simulink model "sppvt_control_model"  (R2024b)
settings: Solver=FixedStepDiscrete  StartTime=0  StopTime=inf  FixedStep=0.05  RelTol=1e-3
undefined symbols (not defined in the file or in its folder): f
libraries: instrumentlib x2
settings Model: Creator=ZhaoY  LastModifiedBy=aiden
settings DataIOCC: ExternalInput=[external_input_data]  SaveFormat=StructureWithTime

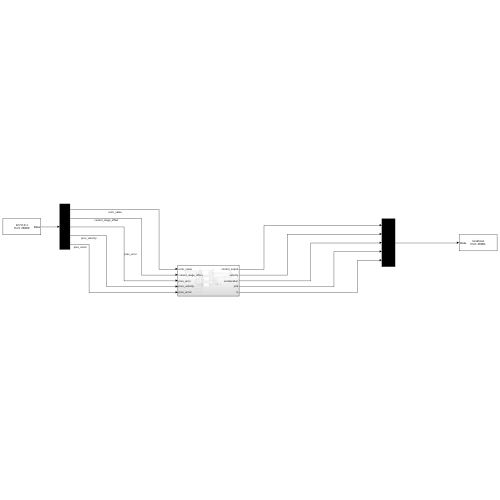
[thumbnail: Simulink's stored preview of the top-level diagram]
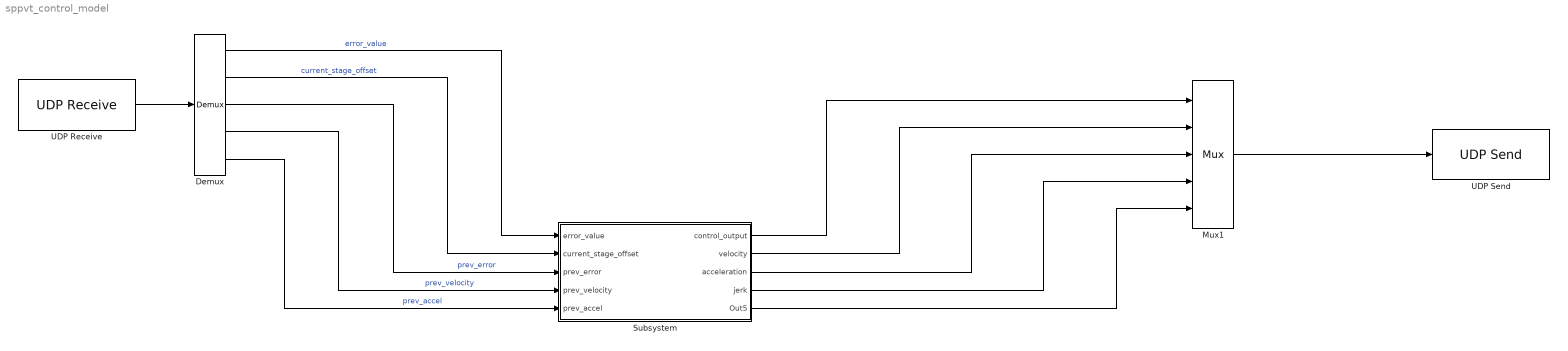
== system sppvt_control_model ==
  Demux : Demux  Outputs=5
  Mux1 : Mux  Inputs=5
  Subsystem : Subsystem
  UDP Receive : instrumentlib/UDP Receive  LocalAddress=127.0.0.1  LocalPort=26000  EnablePortSharing=off  Host=localhost  Port=9091  GetLatestData=on  DataSize=[ 5, 1 ]  DataType=double  ASCIIFormatting=%f,  Terminator=LF  CustomTerminator=10  ByteOrder=little-endian  EnableBlockingMode=on  Timeout=20  SampleTime=-1  SimulateUsing=Interpreted execution
  UDP Send : instrumentlib/UDP Send  Host=localhost  Port=26001  LocalAddress=0.0.0.0  LocalPort=26001  EnablePortSharing=on  OutputDatagramPacketSize=512  ByteOrder=little-endian  EnableBlockingMode=off  SimulateUsing=Interpreted execution
  wires:
  UDP Receive/1 -> Demux/1
  Mux1/1 -> UDP Send/1
  Demux/1 -> Subsystem/1(error_value)  "error_value"
  Demux/2 -> Subsystem/2(current_stage_offset)  "current_stage_offset"
  Demux/3 -> Subsystem/3(prev_error)  "prev_error"
  Demux/4 -> Subsystem/4(prev_velocity)  "prev_velocity"
  Demux/5 -> Subsystem/5(prev_accel)  "prev_accel"
  Subsystem/1(control_output) -> Mux1/1
  Subsystem/2(velocity) -> Mux1/2
  Subsystem/3(acceleration) -> Mux1/3
  Subsystem/4(jerk) -> Mux1/4
  Subsystem/5(Out5) -> Mux1/5

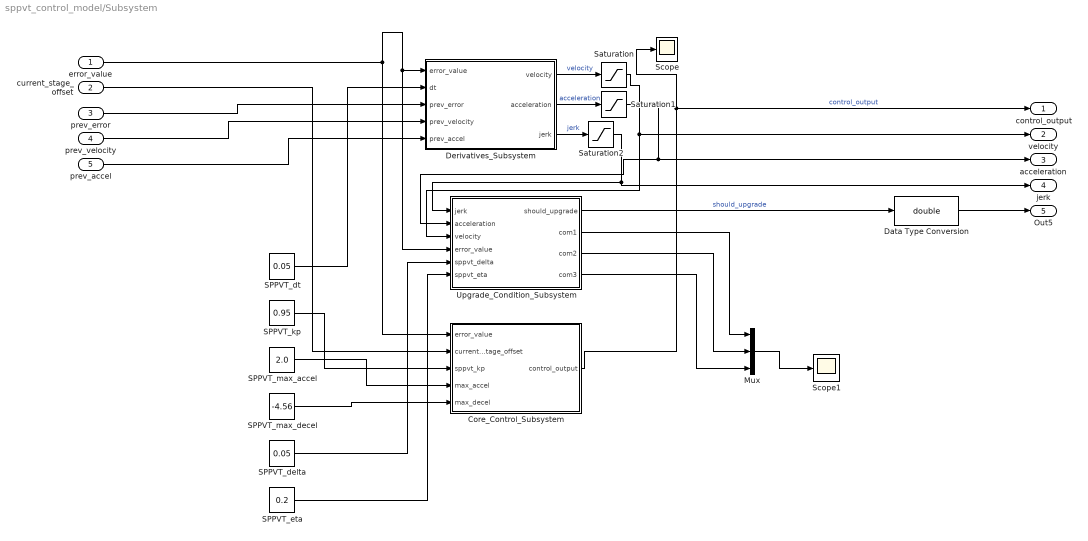
== system sppvt_control_model/Subsystem ==
  error_value : Inport
  current_stage_offset : Inport  Port=2
  prev_error : Inport  Port=3
  prev_velocity : Inport  Port=4
  prev_accel : Inport  Port=5
  Core_Control_Subsystem : Subsystem
  Data Type Conversion : DataTypeConversion  OutDataTypeStr=double  SaturateOnIntegerOverflow=off  RndMeth=Floor
  Derivatives_Subsystem : Subsystem
  Mux : Mux  Inputs=3
  SPPVT_delta : Constant  Value=0.05
  SPPVT_dt : Constant  Value=0.05
  SPPVT_eta : Constant  Value=0.2
  SPPVT_kp : Constant  Value=0.95
  SPPVT_max_accel : Constant  Value=2.0
  SPPVT_max_decel : Constant  Value=-4.56
  Saturation : Saturate  UpperLimit=5000.0  LowerLimit=-5000.0
  Saturation1 : Saturate  UpperLimit=10000.0  LowerLimit=-10000.0
  Saturation2 : Saturate  UpperLimit=20000.0  LowerLimit=-20000.0
  Scope : Scope
  Scope1 : Scope
  Upgrade_Condition_Subsystem : Subsystem
  control_output : Outport
  velocity : Outport  Port=2
  acceleration : Outport  Port=3
  jerk : Outport  Port=4
  Out5 : Outport  Port=5
  wires:
  Upgrade_Condition_Subsystem/2(com1) -> Mux/1
  Derivatives_Subsystem/3(jerk) -> Saturation2/1  "jerk"
  SPPVT_kp/1 -> Core_Control_Subsystem/3(sppvt_kp)
  Derivatives_Subsystem/2(acceleration) -> Saturation1/1  "acceleration"
  Derivatives_Subsystem/1(velocity) -> Saturation/1  "velocity"
  Core_Control_Subsystem/1(control_output) -> control_output/1, Scope/1  "control_output"
  current_stage_offset/1 -> Core_Control_Subsystem/2(current_stage_offset)
  Saturation2/1 -> jerk/1, Upgrade_Condition_Subsystem/1(jerk)
  Data Type Conversion/1 -> Out5/1
  prev_error/1 -> Derivatives_Subsystem/3(prev_error)
  Saturation/1 -> velocity/1, Upgrade_Condition_Subsystem/3(velocity)
  prev_velocity/1 -> Derivatives_Subsystem/4(prev_velocity)
  SPPVT_max_accel/1 -> Core_Control_Subsystem/4(max_accel)
  Upgrade_Condition_Subsystem/1(should_upgrade) -> Data Type Conversion/1  "should_upgrade"
  prev_accel/1 -> Derivatives_Subsystem/5(prev_accel)
  SPPVT_dt/1 -> Derivatives_Subsystem/2(dt)
  Upgrade_Condition_Subsystem/3(com2) -> Mux/2
  SPPVT_eta/1 -> Upgrade_Condition_Subsystem/6(sppvt_eta)
  SPPVT_delta/1 -> Upgrade_Condition_Subsystem/5(sppvt_delta)
  Saturation1/1 -> acceleration/1, Upgrade_Condition_Subsystem/2(acceleration)
  Upgrade_Condition_Subsystem/4(com3) -> Mux/3
  error_value/1 -> Upgrade_Condition_Subsystem/4(error_value), Derivatives_Subsystem/1(error_value), Core_Control_Subsystem/1(error_value)
  Mux/1 -> Scope1/1
  SPPVT_max_decel/1 -> Core_Control_Subsystem/5(max_decel)

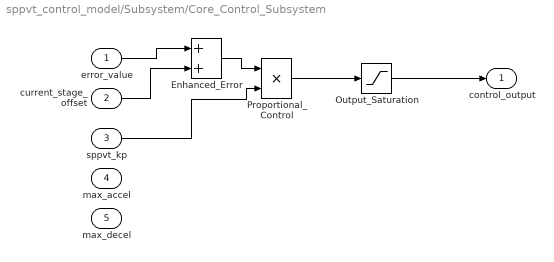
== system sppvt_control_model/Subsystem/Core_Control_Subsystem ==
  error_value : Inport
  current_stage_offset : Inport  Port=2
  sppvt_kp : Inport  Port=3
  max_accel : Inport  Port=4
  max_decel : Inport  Port=5
  Enhanced_Error : Sum
  Output_Saturation : Saturate  UpperLimit=2.0  LowerLimit=-3.0
  Proportional_Control : Product
  control_output : Outport
  wires:
  Proportional_Control/1 -> Output_Saturation/1
  Output_Saturation/1 -> control_output/1
  sppvt_kp/1 -> Proportional_Control/2
  current_stage_offset/1 -> Enhanced_Error/2
  error_value/1 -> Enhanced_Error/1
  Enhanced_Error/1 -> Proportional_Control/1

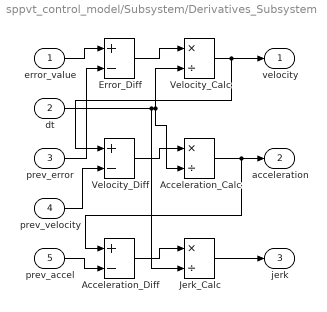
== system sppvt_control_model/Subsystem/Derivatives_Subsystem ==
  error_value : Inport
  dt : Inport  Port=2
  prev_error : Inport  Port=3
  prev_velocity : Inport  Port=4
  prev_accel : Inport  Port=5
  Acceleration_Calc : Product  Inputs=*/
  Acceleration_Diff : Sum  Inputs=+-
  Error_Diff : Sum  Inputs=+-
  Jerk_Calc : Product  Inputs=*/
  Velocity_Calc : Product  Inputs=*/
  Velocity_Diff : Sum  Inputs=+-
  velocity : Outport
  acceleration : Outport  Port=2
  jerk : Outport  Port=3
  wires:
  Velocity_Calc/1 -> Velocity_Diff/1, velocity/1
  Acceleration_Calc/1 -> Acceleration_Diff/1, acceleration/1
  Jerk_Calc/1 -> jerk/1
  error_value/1 -> Error_Diff/1
  prev_error/1 -> Error_Diff/2
  Error_Diff/1 -> Velocity_Calc/1
  prev_accel/1 -> Acceleration_Diff/2
  prev_velocity/1 -> Velocity_Diff/2
  Acceleration_Diff/1 -> Jerk_Calc/1
  dt/1 -> Jerk_Calc/2, Acceleration_Calc/2, Velocity_Calc/2
  Velocity_Diff/1 -> Acceleration_Calc/1

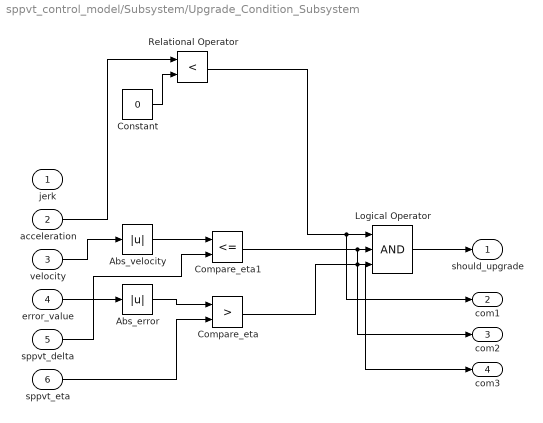
== system sppvt_control_model/Subsystem/Upgrade_Condition_Subsystem ==
  jerk : Inport
  acceleration : Inport  Port=2
  velocity : Inport  Port=3
  error_value : Inport  Port=4
  sppvt_delta : Inport  Port=5
  sppvt_eta : Inport  Port=6
  Abs_error : Abs  SaturateOnIntegerOverflow=off
  Abs_velocity : Abs  SaturateOnIntegerOverflow=off
  Compare_eta : RelationalOperator  Operator=>  OutDataTypeStr=boolean  RndMeth=Simplest  InputSameDT=off
  Compare_eta1 : RelationalOperator  Operator=<=  OutDataTypeStr=boolean  RndMeth=Simplest  InputSameDT=off
  Constant : Constant  Value=0
  Logical Operator : Logic  Inputs=3  AllPortsSameDT=off  OutDataTypeStr=boolean
  Relational Operator : RelationalOperator  Operator=<  OutDataTypeStr=boolean  RndMeth=Simplest  InputSameDT=off
  should_upgrade : Outport
  com1 : Outport  Port=2
  com2 : Outport  Port=3
  com3 : Outport  Port=4
  wires:
  error_value/1 -> Abs_error/1
  Abs_error/1 -> Compare_eta/1
  sppvt_eta/1 -> Compare_eta/2
  acceleration/1 -> Relational Operator/1
  Constant/1 -> Relational Operator/2
  velocity/1 -> Abs_velocity/1
  Abs_velocity/1 -> Compare_eta1/1
  sppvt_delta/1 -> Compare_eta1/2
  Relational Operator/1 -> com1/1, Logical Operator/1
  Compare_eta1/1 -> com2/1, Logical Operator/2
  Compare_eta/1 -> com3/1, Logical Operator/3
  Logical Operator/1 -> should_upgrade/1
